simulink model "PVRobusMPC_final"  (R2018a)
settings: Solver=ode2  StartTime=0.0  StopTime=43200  FixedStep=1  RelTol=1e-3  EnableMultiTasking=on
InitFcn:
  | load PV_model_data
StopFcn:
  | save results Lambda_UV01 T_PV_Reference Tm_f01 Pout01 Tamb Time
  | clear all
  | load results
  | figure
  | subplot(3,1,1)
  | plot(Time./3600,T_PV_Reference,Time./3600,Tm_f01)
  | legend('PV Temperature Reference','PV Temperature')
  | title('MPC Tracking')
  | ylim([350 380])
  | subplot(3,1,2)
  | plot(Time./3600,Lambda_UV01)
  | ylim([250 450])
  | legend('\lambda_U_V')
  | subplot(3,1,3)
  | plot(Time./3600,Pout01)
  | legend('PV Power')
  | xlabel('Time [hours]')
  | ylabel('Watt')
values from neighbouring files (symbols this model uses):
  Global_tilt_Irr_2_2_12_13_5 = [0.000279 0.000786 0.00115 0.00401 0.0047 0.0102 0.011 0.0195 0.0266 0.0299 0.0338 0.0682 ... (2802 elements, 1401x2)]    [PV_model_data.mat]
  Total_light_absorption_in_polystyren = [0.0148235487596 0.0159326919994 0.0170383922491 0.0181406655151 0.0192395277052 0.0203349946285 0.0214270819969 0.0225158054254 0.0236011804327 0.0246832224425 0.0257619467839 0.0264640052027 ... (1151 elements, 1151x1)]    [PV_model_data.mat]
  Total_light_absorption_in_PV_cell_acrylic = [0.0222539070262 0.0239185757929 0.0255780524095 0.0272323791236 0.0288816001883 0.030525761736 0.0321649116541 0.0337990994657 0.0354283762117 0.0370527943369 0.0386724075795 0.0397267002838 ... (1151 elements, 1151x1)]    [PV_model_data.mat]
libraries: mpclib x256
(part 60 of 72)

== matlab function PVRobusMPC_final/4 x 4 x 4 PV Panel 4/4 x 4 PV Panel 5/4 PV Panel 1/PV Panel 2/Photovolatic Panel/PV_Cell_Model ==
  data: Total_light_absorption_in_PV_cell_acrylic parameter; Global_tilt_Irr_2_2_12_13_5 parameter; Total_light_absorption_in_polystyren parameter; Tm_i input; Lambda_UV input; Lambda_IR input; Time input; Tm_f output size=1; QQ output; Tambient input; WS input; VL output
function [Tm_f, QQ, VL] = fcn(Total_light_absorption_in_PV_cell_acrylic, Global_tilt_Irr_2_2_12_13_5, Total_light_absorption_in_polystyren, Tm_i, Lambda_UV, Lambda_IR, Time,Tambient,WS)

IL1 = zeros(1,11);
IL1 = IL1';
LambdaIR_Index = 0;
LambdaUV_Index = 0;
Tm_f =0;
temp_out = 0;

k=1.38e-23; %Boltzman constat J/K
h=6.62617e-34; %Planck constant J.s 
c=3e8; %(m/s) light speed
q=1.60218e-19; %(J) charge of electron
Aj= 148.25; % (cm^2)Junction Area calculated from the dimensions of the module, where length*wedth are 125*125 mm2
M= 4; % number of cells in the BP585 module  From area of module divided by area of one cell
A1=(25.6)^2*1e-4; % Whole area of the module in m^2 (26.1 cm by 26.1 cm)
A=M*Aj*1e-4; % (m^2)Area of the module covered with PV cells 
Beta=pi*65/180; % (deg) tilt angle
segma=5.669*10^(-8); %Stefan_Boltzman W/(m^2K^4)
e_sky_clear = 0.95; %emissivity of the sky in clear wheather conditions
e_g = 0.95; % emissivity of the ground
e_m=0.94; %emissivity of the module which is equale to the emissivity of acrylic and glass
deltT=20; % for clear conditions
dt=1; % Define the step value,
K=Time; % constant equal to the number of seconds of sun exposure, this is equivalent to about 18 mins of sun exposure to same (assumed) solar irraiance 
 
%% Calculating the reference saturation current Ior from the unloaded PV module measurements

Voc = 2.084;	%(V) at reference temperature 26.5 C on 02/02 Module 2 with Acrylic
Isc =4.28; % (A)at reference temperature 26.5 C on 02/02 Module 2 with Acrylic
Rch = Voc/Isc; % (Ohm) Characteristic resistance, this should be found at the characteristic Voc and Isc (ex. Temp = 26.5)
N =1.3812; % Ideality factor for Si-Monocrystalline (reference)
Rs= 0.0377; % (Ohm) Series resistance estimated from the IV curve of M2 covered by accrylic
Tmr = 69.5+273.5; %(K) reference temperature
Ior= Isc/(exp(q*Voc/(M*k*N*Tmr))-1); % (A)Reference saturation current
Eg = 1.12; % (eV) bandgap energy of Si

%% Calculating the heat capacity of the module layers

C_PV=A*2330*677*2e-4; % Heat capacity of the cells (equale to area*raw* specific heat*thickness) source: matweb.com
C_Polystyrene= A*1300*121.7*5e-3; %Heat capacity of the Polystyrene Back supporting board to PV cells 
C_acrylic=A*1470*1190*3.2e-3;% Heat capacity of the Acrylic face over the module

Cm=C_PV+C_Polystyrene+C_acrylic; % Heat capacity of the PV module covered with acrylic


if Lambda_IR<300
    Lambda_IR=300;
elseif Lambda_IR>1700
    Lambda_IR=1700;
end

if Lambda_UV<300
    Lambda_UV=300;
elseif Lambda_UV>1700
    Lambda_UV=1700;
end

 LambdaIR_Index=interp1(Global_tilt_Irr_2_2_12_13_5(:,2),1:1401,Lambda_IR,'nearest');
 LambdaUV_Index=interp1(Global_tilt_Irr_2_2_12_13_5(:,2),1:1401,Lambda_UV,'nearest');

%         LambdaIR_Index=j;
%     end
%     if Lambda_UV==Global_tilt_Irr_2_2_12_13_5(j,2)
%         LambdaUV_Index=j;
%     end
% end


 %% Defining the optical and electrical properties of the used PV module
    U= LambdaIR_Index; %Index for Max. wavelength of IR not to block
%     O=1; % Factor to change the ambient temperauter, this is used to factor Taminet (assumable)to vary the reagion. 
    P=1; % P is assumed number of periods that solar irrandiance is almost same for these periods. 
    Index=0; % the index to take off from maximum Lambda IR that can be absorbed
    D=LambdaUV_Index;%1; % initial value that should be given to D (Index for Max. wavelength of UV to block) 
    Lamda = LambdaIR_Index; % 811; % index at which the maximum absorbed wavelength   
    IQE = 0.69005; % internal quantum efficiency of the cell
    RL = 0.356; % (Ohm) Resistive load (designed and experimentally measured)
    IL1(1,1) = 4;% (A) Load current (experimentally measure)
     
%     Lamda
%% Initializing the matrices

%      Io = NaN;
     wavelength=ones(1451,1);
     Tran = ones(1451,1);
     E=ones(1451,1);
     Photon_flux = ones(1451,1);
     Jph=ones(1451,1);
     Iph = ones(1451,1);
%      Voc = ones;
%      IL = ones;
%      VL = ones;
%      P_out = ones;
     frr =ones(1451,1);
     frr_poly = ones(1451,1);
%      Tm=ones(1,D);
%      hc_free=ones(1,D);
     

IL1(1,1) = 4;% (A) Load current (experimentally measure)

%% Finding the phtonic flux
Tran=Total_light_absorption_in_PV_cell_acrylic(1:U); % Total light transmission considering all layers and bounces through them
wavelength= 1e-9.*Global_tilt_Irr_2_2_12_13_5(1:U,2); % (m) wavelength
E = c.*h./wavelength; % (J) Energy per each wavelength
Photon_flux = Global_tilt_Irr_2_2_12_13_5(1:U,1)./E; % (photons/m2/nm/s) photon flux 

% for w=1 %:1:P*K/dt  
   w=1;

   
    Jph(D:Lamda)= q.*Tran(D:1:Lamda).*Photon_flux(D:Lamda).*IQE; %(Culomb/m2/nm/m/s = A/m2/nm)Short circuit current density 
    Iph(D:Lamda)= Aj.*1e-4.*Jph(D:Lamda); % (A/nm) Photo_generated current 


%% Photonic current per one cell
%    for z=D:1:Lamda
%     Jph(z,1)= q*Tran(z,1)*Photon_flux(z,1)*IQE; %(Culomb/m2/nm/m/s = A/m2/nm)Short circuit current density 
%     Iph (z,1) = Aj*1e-4*Jph(z,1); % (A/nm) Photo_generated current 
%    end
  
  Iph_total =0; % Intializing the current
  
%     for j=D:1:Lamda
        Iph_total = sum(Iph(D:Lamda,1)); % (A) Photonic current
%     end    
  
%% Calculating the input power term to cells
      Irr_total=0;
      
%       for j=D:1:Lamda
           E(D:1:Lamda)=h.*c./(wavelength(D:1:Lamda)); %(J) energy in each wavelength
           Irr_total= sum(Photon_flux(D:1:Lamda,1).*E(D:1:Lamda,1));% (W/m2/nm)Irradiance
%            Irr_total= frr(j,1)+Irr_total; % (W/m^2), this represents the integration to calculate total Irradiance for the specific wavelenght range. 
%       end

      Pin=Irr_total* A; % input power (W) to the module of M cells, each has Aj area in cm^2, A=M*Aj*1e-4    
      
%% Calculating the power input to the Polystyrene backing board
    Irr_poly=0;
    
%     for j=D:1:U % This represents the part of the board covered with cell
         E(D:1:U)=h.*c/(wavelength(D:1:U));
%          frr_poly(j,1)=Photon_flux(j,1)*Total_light_absorption_in_polystyren(j,1)*E(j,1);
         Irr_poly=sum(Photon_flux(D:1:U).*Total_light_absorption_in_polystyren(D:1:U).*E(D:1:U));
%     end

    Ppoly =Irr_poly*(A1-A); % (W) The power produced by the light absorbed by the backing Polystyrene plate

%% Calculating the saturation current using the refernece saturation current method
  
Io= Ior * (Tm_i/Tmr)^3*exp(q*Eg*(1/Tmr-1/Tm_i)/(k*N)); %(A) Saturation current as function of temperature
    
%% Calculating the output power consumed by the load
    nu=0.2; % solver constant
    %This loop is to solve for the load current numberically using Euler method 
    for s=1:1:10% s is counter reflects number of the solver steps needed to reach steady state current at a specific time step
        IL1(s+1) =nu*IL1(s)+(1-nu)*( N*k*Tm_i/(q*(RL/M+Rs))*log((Iph_total-IL1(s))/(Io)+1));
    end
%     IL1
    IL = IL1(end); % (V) Stabalized Output current passes the resistive load (0.3525 Ohm)in one time step
%     IL1 = IL1(end);  % setting a new initial load current for the next time step
    VL =  IL *RL; %Load voltage, or Iph_total-Io(w,1)*(exp(q*VL(w,1)/(N*k*Tm(w,1))-1)); %(A) Output current
   
%     P_out =real(VL*IL); %(W) Output power across the load 
   P_out=real(VL*IL);
   P_out=P_out(1);
   QQ=VL.*IL;
%  P_out(w,1)=0; % In case of open circuit condition

%% Calculating the output power in case of tracking the MPP
%      
%      Voc(w,1) = N*k*Tm(w,1)/q*log(Iph_total/Io(w,1)+1) ;  % (V) open circuit voltage
% 
%      Vocn(w,1)=q/(N*k*Tm(w,1))*Voc(w,1); % Normalized open circuit voltage
% 
%      Cff (w,1) = (Vocn(w,1)-log(Vocn(w,1)+0.72))/(Vocn(w,1)+1); % Filling factor
%               
%      rs=Rs/Rch; % ratio
%      
%      Cffn(w,1)=Cff(w,1)*(1-rs); % impact of the series resistance on the IV curve
%      
%     P_out(w,1)=M*Cffn(w,1)*Iph_total*Voc(w,1); % (W) output power of the module
      
%% Defining the terms of heat transfer


 
  hc_forced = 3.3*WS+6.5; % (W/(m^2.K)) Sharples windward relation to calculated hc_forced from the averaged wind speed 
    
  hc_free=1.31*(Tm_i-Tambient)^(1/3); % (W/(M^2.K)) Heat transfer coefficient due to air cooling on top surface and no wind
     
    Tsky=Tambient-deltT; % (K) Sky temperature
    %Tsky=Tambient; % (K) for overcast conditions
    Tground=Tambient; %(K) Ground temperature
     
%% Solving the 1st order nonlinear differenctial equation using Euler method
     Tm_f=Tm_i+dt.*(1/Cm*(segma*A*(((1+cos(Beta)/2)*e_sky_clear*(Tsky)^(4))+((1-cos(Beta))/2*e_g*(Tground)^(4))-(e_m*(Tm_i)^(4)))+ Ppoly + Pin -P_out-A.*(hc_forced^3+hc_free^3).^(1/3).*(Tm_i-Tambient))); %(K)Finding the module Temp

== matlab function PVRobusMPC_final/4 x 4 x 4 PV Panel 4/4 x 4 PV Panel 5/4 PV Panel 1/PV Panel 3/Photovolatic Panel/PV_Cell_Model ==
  data: Total_light_absorption_in_PV_cell_acrylic parameter; Global_tilt_Irr_2_2_12_13_5 parameter; Total_light_absorption_in_polystyren parameter; Tm_i input; Lambda_UV input; Lambda_IR input; Time input; Tm_f output size=1; QQ output; Tambient input; WS input; VL output
function [Tm_f, QQ, VL] = fcn(Total_light_absorption_in_PV_cell_acrylic, Global_tilt_Irr_2_2_12_13_5, Total_light_absorption_in_polystyren, Tm_i, Lambda_UV, Lambda_IR, Time,Tambient,WS)

IL1 = zeros(1,11);
IL1 = IL1';
LambdaIR_Index = 0;
LambdaUV_Index = 0;
Tm_f =0;
temp_out = 0;

k=1.38e-23; %Boltzman constat J/K
h=6.62617e-34; %Planck constant J.s 
c=3e8; %(m/s) light speed
q=1.60218e-19; %(J) charge of electron
Aj= 148.25; % (cm^2)Junction Area calculated from the dimensions of the module, where length*wedth are 125*125 mm2
M= 4; % number of cells in the BP585 module  From area of module divided by area of one cell
A1=(25.6)^2*1e-4; % Whole area of the module in m^2 (26.1 cm by 26.1 cm)
A=M*Aj*1e-4; % (m^2)Area of the module covered with PV cells 
Beta=pi*65/180; % (deg) tilt angle
segma=5.669*10^(-8); %Stefan_Boltzman W/(m^2K^4)
e_sky_clear = 0.95; %emissivity of the sky in clear wheather conditions
e_g = 0.95; % emissivity of the ground
e_m=0.94; %emissivity of the module which is equale to the emissivity of acrylic and glass
deltT=20; % for clear conditions
dt=1; % Define the step value,
K=Time; % constant equal to the number of seconds of sun exposure, this is equivalent to about 18 mins of sun exposure to same (assumed) solar irraiance 
 
%% Calculating the reference saturation current Ior from the unloaded PV module measurements

Voc = 2.084;	%(V) at reference temperature 26.5 C on 02/02 Module 2 with Acrylic
Isc =4.28; % (A)at reference temperature 26.5 C on 02/02 Module 2 with Acrylic
Rch = Voc/Isc; % (Ohm) Characteristic resistance, this should be found at the characteristic Voc and Isc (ex. Temp = 26.5)
N =1.3812; % Ideality factor for Si-Monocrystalline (reference)
Rs= 0.0377; % (Ohm) Series resistance estimated from the IV curve of M2 covered by accrylic
Tmr = 69.5+273.5; %(K) reference temperature
Ior= Isc/(exp(q*Voc/(M*k*N*Tmr))-1); % (A)Reference saturation current
Eg = 1.12; % (eV) bandgap energy of Si

%% Calculating the heat capacity of the module layers

C_PV=A*2330*677*2e-4; % Heat capacity of the cells (equale to area*raw* specific heat*thickness) source: matweb.com
C_Polystyrene= A*1300*121.7*5e-3; %Heat capacity of the Polystyrene Back supporting board to PV cells 
C_acrylic=A*1470*1190*3.2e-3;% Heat capacity of the Acrylic face over the module

Cm=C_PV+C_Polystyrene+C_acrylic; % Heat capacity of the PV module covered with acrylic


if Lambda_IR<300
    Lambda_IR=300;
elseif Lambda_IR>1700
    Lambda_IR=1700;
end

if Lambda_UV<300
    Lambda_UV=300;
elseif Lambda_UV>1700
    Lambda_UV=1700;
end

 LambdaIR_Index=interp1(Global_tilt_Irr_2_2_12_13_5(:,2),1:1401,Lambda_IR,'nearest');
 LambdaUV_Index=interp1(Global_tilt_Irr_2_2_12_13_5(:,2),1:1401,Lambda_UV,'nearest');

%         LambdaIR_Index=j;
%     end
%     if Lambda_UV==Global_tilt_Irr_2_2_12_13_5(j,2)
%         LambdaUV_Index=j;
%     end
% end


 %% Defining the optical and electrical properties of the used PV module
    U= LambdaIR_Index; %Index for Max. wavelength of IR not to block
%     O=1; % Factor to change the ambient temperauter, this is used to factor Taminet (assumable)to vary the reagion. 
    P=1; % P is assumed number of periods that solar irrandiance is almost same for these periods. 
    Index=0; % the index to take off from maximum Lambda IR that can be absorbed
    D=LambdaUV_Index;%1; % initial value that should be given to D (Index for Max. wavelength of UV to block) 
    Lamda = LambdaIR_Index; % 811; % index at which the maximum absorbed wavelength   
    IQE = 0.69005; % internal quantum efficiency of the cell
    RL = 0.356; % (Ohm) Resistive load (designed and experimentally measured)
    IL1(1,1) = 4;% (A) Load current (experimentally measure)
     
%     Lamda
%% Initializing the matrices

%      Io = NaN;
     wavelength=ones(1451,1);
     Tran = ones(1451,1);
     E=ones(1451,1);
     Photon_flux = ones(1451,1);
     Jph=ones(1451,1);
     Iph = ones(1451,1);
%      Voc = ones;
%      IL = ones;
%      VL = ones;
%      P_out = ones;
     frr =ones(1451,1);
     frr_poly = ones(1451,1);
%      Tm=ones(1,D);
%      hc_free=ones(1,D);
     

IL1(1,1) = 4;% (A) Load current (experimentally measure)

%% Finding the phtonic flux
Tran=Total_light_absorption_in_PV_cell_acrylic(1:U); % Total light transmission considering all layers and bounces through them
wavelength= 1e-9.*Global_tilt_Irr_2_2_12_13_5(1:U,2); % (m) wavelength
E = c.*h./wavelength; % (J) Energy per each wavelength
Photon_flux = Global_tilt_Irr_2_2_12_13_5(1:U,1)./E; % (photons/m2/nm/s) photon flux 

% for w=1 %:1:P*K/dt  
   w=1;

   
    Jph(D:Lamda)= q.*Tran(D:1:Lamda).*Photon_flux(D:Lamda).*IQE; %(Culomb/m2/nm/m/s = A/m2/nm)Short circuit current density 
    Iph(D:Lamda)= Aj.*1e-4.*Jph(D:Lamda); % (A/nm) Photo_generated current 


%% Photonic current per one cell
%    for z=D:1:Lamda
%     Jph(z,1)= q*Tran(z,1)*Photon_flux(z,1)*IQE; %(Culomb/m2/nm/m/s = A/m2/nm)Short circuit current density 
%     Iph (z,1) = Aj*1e-4*Jph(z,1); % (A/nm) Photo_generated current 
%    end
  
  Iph_total =0; % Intializing the current
  
%     for j=D:1:Lamda
        Iph_total = sum(Iph(D:Lamda,1)); % (A) Photonic current
%     end    
  
%% Calculating the input power term to cells
      Irr_total=0;
      
%       for j=D:1:Lamda
           E(D:1:Lamda)=h.*c./(wavelength(D:1:Lamda)); %(J) energy in each wavelength
           Irr_total= sum(Photon_flux(D:1:Lamda,1).*E(D:1:Lamda,1));% (W/m2/nm)Irradiance
%            Irr_total= frr(j,1)+Irr_total; % (W/m^2), this represents the integration to calculate total Irradiance for the specific wavelenght range. 
%       end

      Pin=Irr_total* A; % input power (W) to the module of M cells, each has Aj area in cm^2, A=M*Aj*1e-4    
      
%% Calculating the power input to the Polystyrene backing board
    Irr_poly=0;
    
%     for j=D:1:U % This represents the part of the board covered with cell
         E(D:1:U)=h.*c/(wavelength(D:1:U));
%          frr_poly(j,1)=Photon_flux(j,1)*Total_light_absorption_in_polystyren(j,1)*E(j,1);
         Irr_poly=sum(Photon_flux(D:1:U).*Total_light_absorption_in_polystyren(D:1:U).*E(D:1:U));
%     end

    Ppoly =Irr_poly*(A1-A); % (W) The power produced by the light absorbed by the backing Polystyrene plate

%% Calculating the saturation current using the refernece saturation current method
  
Io= Ior * (Tm_i/Tmr)^3*exp(q*Eg*(1/Tmr-1/Tm_i)/(k*N)); %(A) Saturation current as function of temperature
    
%% Calculating the output power consumed by the load
    nu=0.2; % solver constant
    %This loop is to solve for the load current numberically using Euler method 
    for s=1:1:10% s is counter reflects number of the solver steps needed to reach steady state current at a specific time step
        IL1(s+1) =nu*IL1(s)+(1-nu)*( N*k*Tm_i/(q*(RL/M+Rs))*log((Iph_total-IL1(s))/(Io)+1));
    end
%     IL1
    IL = IL1(end); % (V) Stabalized Output current passes the resistive load (0.3525 Ohm)in one time step
%     IL1 = IL1(end);  % setting a new initial load current for the next time step
    VL =  IL *RL; %Load voltage, or Iph_total-Io(w,1)*(exp(q*VL(w,1)/(N*k*Tm(w,1))-1)); %(A) Output current
   
%     P_out =real(VL*IL); %(W) Output power across the load 
   P_out=real(VL*IL);
   P_out=P_out(1);
   QQ=VL.*IL;
%  P_out(w,1)=0; % In case of open circuit condition

%% Calculating the output power in case of tracking the MPP
%      
%      Voc(w,1) = N*k*Tm(w,1)/q*log(Iph_total/Io(w,1)+1) ;  % (V) open circuit voltage
% 
%      Vocn(w,1)=q/(N*k*Tm(w,1))*Voc(w,1); % Normalized open circuit voltage
% 
%      Cff (w,1) = (Vocn(w,1)-log(Vocn(w,1)+0.72))/(Vocn(w,1)+1); % Filling factor
%               
%      rs=Rs/Rch; % ratio
%      
%      Cffn(w,1)=Cff(w,1)*(1-rs); % impact of the series resistance on the IV curve
%      
%     P_out(w,1)=M*Cffn(w,1)*Iph_total*Voc(w,1); % (W) output power of the module
      
%% Defining the terms of heat transfer


 
  hc_forced = 3.3*WS+6.5; % (W/(m^2.K)) Sharples windward relation to calculated hc_forced from the averaged wind speed 
    
  hc_free=1.31*(Tm_i-Tambient)^(1/3); % (W/(M^2.K)) Heat transfer coefficient due to air cooling on top surface and no wind
     
    Tsky=Tambient-deltT; % (K) Sky temperature
    %Tsky=Tambient; % (K) for overcast conditions
    Tground=Tambient; %(K) Ground temperature
     
%% Solving the 1st order nonlinear differenctial equation using Euler method
     Tm_f=Tm_i+dt.*(1/Cm*(segma*A*(((1+cos(Beta)/2)*e_sky_clear*(Tsky)^(4))+((1-cos(Beta))/2*e_g*(Tground)^(4))-(e_m*(Tm_i)^(4)))+ Ppoly + Pin -P_out-A.*(hc_forced^3+hc_free^3).^(1/3).*(Tm_i-Tambient))); %(K)Finding the module Temp

== matlab function PVRobusMPC_final/4 x 4 x 4 PV Panel 4/4 x 4 PV Panel 5/4 PV Panel 1/PV Panel 4/Photovolatic Panel/PV_Cell_Model ==
  data: Total_light_absorption_in_PV_cell_acrylic parameter; Global_tilt_Irr_2_2_12_13_5 parameter; Total_light_absorption_in_polystyren parameter; Tm_i input; Lambda_UV input; Lambda_IR input; Time input; Tm_f output size=1; QQ output; Tambient input; WS input; VL output
function [Tm_f, QQ, VL] = fcn(Total_light_absorption_in_PV_cell_acrylic, Global_tilt_Irr_2_2_12_13_5, Total_light_absorption_in_polystyren, Tm_i, Lambda_UV, Lambda_IR, Time,Tambient,WS)

IL1 = zeros(1,11);
IL1 = IL1';
LambdaIR_Index = 0;
LambdaUV_Index = 0;
Tm_f =0;
temp_out = 0;

k=1.38e-23; %Boltzman constat J/K
h=6.62617e-34; %Planck constant J.s 
c=3e8; %(m/s) light speed
q=1.60218e-19; %(J) charge of electron
Aj= 148.25; % (cm^2)Junction Area calculated from the dimensions of the module, where length*wedth are 125*125 mm2
M= 4; % number of cells in the BP585 module  From area of module divided by area of one cell
A1=(25.6)^2*1e-4; % Whole area of the module in m^2 (26.1 cm by 26.1 cm)
A=M*Aj*1e-4; % (m^2)Area of the module covered with PV cells 
Beta=pi*65/180; % (deg) tilt angle
segma=5.669*10^(-8); %Stefan_Boltzman W/(m^2K^4)
e_sky_clear = 0.95; %emissivity of the sky in clear wheather conditions
e_g = 0.95; % emissivity of the ground
e_m=0.94; %emissivity of the module which is equale to the emissivity of acrylic and glass
deltT=20; % for clear conditions
dt=1; % Define the step value,
K=Time; % constant equal to the number of seconds of sun exposure, this is equivalent to about 18 mins of sun exposure to same (assumed) solar irraiance 
 
%% Calculating the reference saturation current Ior from the unloaded PV module measurements

Voc = 2.084;	%(V) at reference temperature 26.5 C on 02/02 Module 2 with Acrylic
Isc =4.28; % (A)at reference temperature 26.5 C on 02/02 Module 2 with Acrylic
Rch = Voc/Isc; % (Ohm) Characteristic resistance, this should be found at the characteristic Voc and Isc (ex. Temp = 26.5)
N =1.3812; % Ideality factor for Si-Monocrystalline (reference)
Rs= 0.0377; % (Ohm) Series resistance estimated from the IV curve of M2 covered by accrylic
Tmr = 69.5+273.5; %(K) reference temperature
Ior= Isc/(exp(q*Voc/(M*k*N*Tmr))-1); % (A)Reference saturation current
Eg = 1.12; % (eV) bandgap energy of Si

%% Calculating the heat capacity of the module layers

C_PV=A*2330*677*2e-4; % Heat capacity of the cells (equale to area*raw* specific heat*thickness) source: matweb.com
C_Polystyrene= A*1300*121.7*5e-3; %Heat capacity of the Polystyrene Back supporting board to PV cells 
C_acrylic=A*1470*1190*3.2e-3;% Heat capacity of the Acrylic face over the module

Cm=C_PV+C_Polystyrene+C_acrylic; % Heat capacity of the PV module covered with acrylic


if Lambda_IR<300
    Lambda_IR=300;
elseif Lambda_IR>1700
    Lambda_IR=1700;
end

if Lambda_UV<300
    Lambda_UV=300;
elseif Lambda_UV>1700
    Lambda_UV=1700;
end

 LambdaIR_Index=interp1(Global_tilt_Irr_2_2_12_13_5(:,2),1:1401,Lambda_IR,'nearest');
 LambdaUV_Index=interp1(Global_tilt_Irr_2_2_12_13_5(:,2),1:1401,Lambda_UV,'nearest');

%         LambdaIR_Index=j;
%     end
%     if Lambda_UV==Global_tilt_Irr_2_2_12_13_5(j,2)
%         LambdaUV_Index=j;
%     end
% end


 %% Defining the optical and electrical properties of the used PV module
    U= LambdaIR_Index; %Index for Max. wavelength of IR not to block
%     O=1; % Factor to change the ambient temperauter, this is used to factor Taminet (assumable)to vary the reagion. 
    P=1; % P is assumed number of periods that solar irrandiance is almost same for these periods. 
    Index=0; % the index to take off from maximum Lambda IR that can be absorbed
    D=LambdaUV_Index;%1; % initial value that should be given to D (Index for Max. wavelength of UV to block) 
    Lamda = LambdaIR_Index; % 811; % index at which the maximum absorbed wavelength   
    IQE = 0.69005; % internal quantum efficiency of the cell
    RL = 0.356; % (Ohm) Resistive load (designed and experimentally measured)
    IL1(1,1) = 4;% (A) Load current (experimentally measure)
     
%     Lamda
%% Initializing the matrices

%      Io = NaN;
     wavelength=ones(1451,1);
     Tran = ones(1451,1);
     E=ones(1451,1);
     Photon_flux = ones(1451,1);
     Jph=ones(1451,1);
     Iph = ones(1451,1);
%      Voc = ones;
%      IL = ones;
%      VL = ones;
%      P_out = ones;
     frr =ones(1451,1);
     frr_poly = ones(1451,1);
%      Tm=ones(1,D);
%      hc_free=ones(1,D);
     

IL1(1,1) = 4;% (A) Load current (experimentally measure)

%% Finding the phtonic flux
Tran=Total_light_absorption_in_PV_cell_acrylic(1:U); % Total light transmission considering all layers and bounces through them
wavelength= 1e-9.*Global_tilt_Irr_2_2_12_13_5(1:U,2); % (m) wavelength
E = c.*h./wavelength; % (J) Energy per each wavelength
Photon_flux = Global_tilt_Irr_2_2_12_13_5(1:U,1)./E; % (photons/m2/nm/s) photon flux 

% for w=1 %:1:P*K/dt  
   w=1;

   
    Jph(D:Lamda)= q.*Tran(D:1:Lamda).*Photon_flux(D:Lamda).*IQE; %(Culomb/m2/nm/m/s = A/m2/nm)Short circuit current density 
    Iph(D:Lamda)= Aj.*1e-4.*Jph(D:Lamda); % (A/nm) Photo_generated current 


%% Photonic current per one cell
%    for z=D:1:Lamda
%     Jph(z,1)= q*Tran(z,1)*Photon_flux(z,1)*IQE; %(Culomb/m2/nm/m/s = A/m2/nm)Short circuit current density 
%     Iph (z,1) = Aj*1e-4*Jph(z,1); % (A/nm) Photo_generated current 
%    end
  
  Iph_total =0; % Intializing the current
  
%     for j=D:1:Lamda
        Iph_total = sum(Iph(D:Lamda,1)); % (A) Photonic current
%     end    
  
%% Calculating the input power term to cells
      Irr_total=0;
      
%       for j=D:1:Lamda
           E(D:1:Lamda)=h.*c./(wavelength(D:1:Lamda)); %(J) energy in each wavelength
           Irr_total= sum(Photon_flux(D:1:Lamda,1).*E(D:1:Lamda,1));% (W/m2/nm)Irradiance
%            Irr_total= frr(j,1)+Irr_total; % (W/m^2), this represents the integration to calculate total Irradiance for the specific wavelenght range. 
%       end

      Pin=Irr_total* A; % input power (W) to the module of M cells, each has Aj area in cm^2, A=M*Aj*1e-4    
      
%% Calculating the power input to the Polystyrene backing board
    Irr_poly=0;
    
%     for j=D:1:U % This represents the part of the board covered with cell
         E(D:1:U)=h.*c/(wavelength(D:1:U));
%          frr_poly(j,1)=Photon_flux(j,1)*Total_light_absorption_in_polystyren(j,1)*E(j,1);
         Irr_poly=sum(Photon_flux(D:1:U).*Total_light_absorption_in_polystyren(D:1:U).*E(D:1:U));
%     end

    Ppoly =Irr_poly*(A1-A); % (W) The power produced by the light absorbed by the backing Polystyrene plate

%% Calculating the saturation current using the refernece saturation current method
  
Io= Ior * (Tm_i/Tmr)^3*exp(q*Eg*(1/Tmr-1/Tm_i)/(k*N)); %(A) Saturation current as function of temperature
    
%% Calculating the output power consumed by the load
    nu=0.2; % solver constant
    %This loop is to solve for the load current numberically using Euler method 
    for s=1:1:10% s is counter reflects number of the solver steps needed to reach steady state current at a specific time step
        IL1(s+1) =nu*IL1(s)+(1-nu)*( N*k*Tm_i/(q*(RL/M+Rs))*log((Iph_total-IL1(s))/(Io)+1));
    end
%     IL1
    IL = IL1(end); % (V) Stabalized Output current passes the resistive load (0.3525 Ohm)in one time step
%     IL1 = IL1(end);  % setting a new initial load current for the next time step
    VL =  IL *RL; %Load voltage, or Iph_total-Io(w,1)*(exp(q*VL(w,1)/(N*k*Tm(w,1))-1)); %(A) Output current
   
%     P_out =real(VL*IL); %(W) Output power across the load 
   P_out=real(VL*IL);
   P_out=P_out(1);
   QQ=VL.*IL;
%  P_out(w,1)=0; % In case of open circuit condition

%% Calculating the output power in case of tracking the MPP
%      
%      Voc(w,1) = N*k*Tm(w,1)/q*log(Iph_total/Io(w,1)+1) ;  % (V) open circuit voltage
% 
%      Vocn(w,1)=q/(N*k*Tm(w,1))*Voc(w,1); % Normalized open circuit voltage
% 
%      Cff (w,1) = (Vocn(w,1)-log(Vocn(w,1)+0.72))/(Vocn(w,1)+1); % Filling factor
%               
%      rs=Rs/Rch; % ratio
%      
%      Cffn(w,1)=Cff(w,1)*(1-rs); % impact of the series resistance on the IV curve
%      
%     P_out(w,1)=M*Cffn(w,1)*Iph_total*Voc(w,1); % (W) output power of the module
      
%% Defining the terms of heat transfer


 
  hc_forced = 3.3*WS+6.5; % (W/(m^2.K)) Sharples windward relation to calculated hc_forced from the averaged wind speed 
    
  hc_free=1.31*(Tm_i-Tambient)^(1/3); % (W/(M^2.K)) Heat transfer coefficient due to air cooling on top surface and no wind
     
    Tsky=Tambient-deltT; % (K) Sky temperature
    %Tsky=Tambient; % (K) for overcast conditions
    Tground=Tambient; %(K) Ground temperature
     
%% Solving the 1st order nonlinear differenctial equation using Euler method
     Tm_f=Tm_i+dt.*(1/Cm*(segma*A*(((1+cos(Beta)/2)*e_sky_clear*(Tsky)^(4))+((1-cos(Beta))/2*e_g*(Tground)^(4))-(e_m*(Tm_i)^(4)))+ Ppoly + Pin -P_out-A.*(hc_forced^3+hc_free^3).^(1/3).*(Tm_i-Tambient))); %(K)Finding the module Temp

== matlab function PVRobusMPC_final/4 x 4 x 4 PV Panel 4/4 x 4 PV Panel 5/4 PV Panel 2/PV Panel 5/Photovolatic Panel/PV_Cell_Model ==
  data: Total_light_absorption_in_PV_cell_acrylic parameter; Global_tilt_Irr_2_2_12_13_5 parameter; Total_light_absorption_in_polystyren parameter; Tm_i input; Lambda_UV input; Lambda_IR input; Time input; Tm_f output size=1; QQ output; Tambient input; WS input; VL output
function [Tm_f, QQ, VL] = fcn(Total_light_absorption_in_PV_cell_acrylic, Global_tilt_Irr_2_2_12_13_5, Total_light_absorption_in_polystyren, Tm_i, Lambda_UV, Lambda_IR, Time,Tambient,WS)

IL1 = zeros(1,11);
IL1 = IL1';
LambdaIR_Index = 0;
LambdaUV_Index = 0;
Tm_f =0;
temp_out = 0;

k=1.38e-23; %Boltzman constat J/K
h=6.62617e-34; %Planck constant J.s 
c=3e8; %(m/s) light speed
q=1.60218e-19; %(J) charge of electron
Aj= 148.25; % (cm^2)Junction Area calculated from the dimensions of the module, where length*wedth are 125*125 mm2
M= 4; % number of cells in the BP585 module  From area of module divided by area of one cell
A1=(25.6)^2*1e-4; % Whole area of the module in m^2 (26.1 cm by 26.1 cm)
A=M*Aj*1e-4; % (m^2)Area of the module covered with PV cells 
Beta=pi*65/180; % (deg) tilt angle
segma=5.669*10^(-8); %Stefan_Boltzman W/(m^2K^4)
e_sky_clear = 0.95; %emissivity of the sky in clear wheather conditions
e_g = 0.95; % emissivity of the ground
e_m=0.94; %emissivity of the module which is equale to the emissivity of acrylic and glass
deltT=20; % for clear conditions
dt=1; % Define the step value,
K=Time; % constant equal to the number of seconds of sun exposure, this is equivalent to about 18 mins of sun exposure to same (assumed) solar irraiance 
 
%% Calculating the reference saturation current Ior from the unloaded PV module measurements

Voc = 2.084;	%(V) at reference temperature 26.5 C on 02/02 Module 2 with Acrylic
Isc =4.28; % (A)at reference temperature 26.5 C on 02/02 Module 2 with Acrylic
Rch = Voc/Isc; % (Ohm) Characteristic resistance, this should be found at the characteristic Voc and Isc (ex. Temp = 26.5)
N =1.3812; % Ideality factor for Si-Monocrystalline (reference)
Rs= 0.0377; % (Ohm) Series resistance estimated from the IV curve of M2 covered by accrylic
Tmr = 69.5+273.5; %(K) reference temperature
Ior= Isc/(exp(q*Voc/(M*k*N*Tmr))-1); % (A)Reference saturation current
Eg = 1.12; % (eV) bandgap energy of Si

%% Calculating the heat capacity of the module layers

C_PV=A*2330*677*2e-4; % Heat capacity of the cells (equale to area*raw* specific heat*thickness) source: matweb.com
C_Polystyrene= A*1300*121.7*5e-3; %Heat capacity of the Polystyrene Back supporting board to PV cells 
C_acrylic=A*1470*1190*3.2e-3;% Heat capacity of the Acrylic face over the module

Cm=C_PV+C_Polystyrene+C_acrylic; % Heat capacity of the PV module covered with acrylic


if Lambda_IR<300
    Lambda_IR=300;
elseif Lambda_IR>1700
    Lambda_IR=1700;
end

if Lambda_UV<300
    Lambda_UV=300;
elseif Lambda_UV>1700
    Lambda_UV=1700;
end

 LambdaIR_Index=interp1(Global_tilt_Irr_2_2_12_13_5(:,2),1:1401,Lambda_IR,'nearest');
 LambdaUV_Index=interp1(Global_tilt_Irr_2_2_12_13_5(:,2),1:1401,Lambda_UV,'nearest');

%         LambdaIR_Index=j;
%     end
%     if Lambda_UV==Global_tilt_Irr_2_2_12_13_5(j,2)
%         LambdaUV_Index=j;
%     end
% end


 %% Defining the optical and electrical properties of the used PV module
    U= LambdaIR_Index; %Index for Max. wavelength of IR not to block
%     O=1; % Factor to change the ambient temperauter, this is used to factor Taminet (assumable)to vary the reagion. 
    P=1; % P is assumed number of periods that solar irrandiance is almost same for these periods. 
    Index=0; % the index to take off from maximum Lambda IR that can be absorbed
    D=LambdaUV_Index;%1; % initial value that should be given to D (Index for Max. wavelength of UV to block) 
    Lamda = LambdaIR_Index; % 811; % index at which the maximum absorbed wavelength   
    IQE = 0.69005; % internal quantum efficiency of the cell
    RL = 0.356; % (Ohm) Resistive load (designed and experimentally measured)
    IL1(1,1) = 4;% (A) Load current (experimentally measure)
     
%     Lamda
%% Initializing the matrices

%      Io = NaN;
     wavelength=ones(1451,1);
     Tran = ones(1451,1);
     E=ones(1451,1);
     Photon_flux = ones(1451,1);
     Jph=ones(1451,1);
     Iph = ones(1451,1);
%      Voc = ones;
%      IL = ones;
%      VL = ones;
%      P_out = ones;
     frr =ones(1451,1);
     frr_poly = ones(1451,1);
%      Tm=ones(1,D);
%      hc_free=ones(1,D);
     

IL1(1,1) = 4;% (A) Load current (experimentally measure)

%% Finding the phtonic flux
Tran=Total_light_absorption_in_PV_cell_acrylic(1:U); % Total light transmission considering all layers and bounces through them
wavelength= 1e-9.*Global_tilt_Irr_2_2_12_13_5(1:U,2); % (m) wavelength
E = c.*h./wavelength; % (J) Energy per each wavelength
Photon_flux = Global_tilt_Irr_2_2_12_13_5(1:U,1)./E; % (photons/m2/nm/s) photon flux 

% for w=1 %:1:P*K/dt  
   w=1;

   
    Jph(D:Lamda)= q.*Tran(D:1:Lamda).*Photon_flux(D:Lamda).*IQE; %(Culomb/m2/nm/m/s = A/m2/nm)Short circuit current density 
    Iph(D:Lamda)= Aj.*1e-4.*Jph(D:Lamda); % (A/nm) Photo_generated current 


%% Photonic current per one cell
%    for z=D:1:Lamda
%     Jph(z,1)= q*Tran(z,1)*Photon_flux(z,1)*IQE; %(Culomb/m2/nm/m/s = A/m2/nm)Short circuit current density 
%     Iph (z,1) = Aj*1e-4*Jph(z,1); % (A/nm) Photo_generated current 
%    end
  
  Iph_total =0; % Intializing the current
  
%     for j=D:1:Lamda
        Iph_total = sum(Iph(D:Lamda,1)); % (A) Photonic current
%     end    
  
%% Calculating the input power term to cells
      Irr_total=0;
      
%       for j=D:1:Lamda
           E(D:1:Lamda)=h.*c./(wavelength(D:1:Lamda)); %(J) energy in each wavelength
           Irr_total= sum(Photon_flux(D:1:Lamda,1).*E(D:1:Lamda,1));% (W/m2/nm)Irradiance
%            Irr_total= frr(j,1)+Irr_total; % (W/m^2), this represents the integration to calculate total Irradiance for the specific wavelenght range. 
%       end

      Pin=Irr_total* A; % input power (W) to the module of M cells, each has Aj area in cm^2, A=M*Aj*1e-4    
      
%% Calculating the power input to the Polystyrene backing board
    Irr_poly=0;
    
%     for j=D:1:U % This represents the part of the board covered with cell
         E(D:1:U)=h.*c/(wavelength(D:1:U));
%          frr_poly(j,1)=Photon_flux(j,1)*Total_light_absorption_in_polystyren(j,1)*E(j,1);
         Irr_poly=sum(Photon_flux(D:1:U).*Total_light_absorption_in_polystyren(D:1:U).*E(D:1:U));
%     end

    Ppoly =Irr_poly*(A1-A); % (W) The power produced by the light absorbed by the backing Polystyrene plate

%% Calculating the saturation current using the refernece saturation current method
  
Io= Ior * (Tm_i/Tmr)^3*exp(q*Eg*(1/Tmr-1/Tm_i)/(k*N)); %(A) Saturation current as function of temperature
    
%% Calculating the output power consumed by the load
    nu=0.2; % solver constant
    %This loop is to solve for the load current numberically using Euler method 
    for s=1:1:10% s is counter reflects number of the solver steps needed to reach steady state current at a specific time step
        IL1(s+1) =nu*IL1(s)+(1-nu)*( N*k*Tm_i/(q*(RL/M+Rs))*log((Iph_total-IL1(s))/(Io)+1));
    end
%     IL1
    IL = IL1(end); % (V) Stabalized Output current passes the resistive load (0.3525 Ohm)in one time step
%     IL1 = IL1(end);  % setting a new initial load current for the next time step
    VL =  IL *RL; %Load voltage, or Iph_total-Io(w,1)*(exp(q*VL(w,1)/(N*k*Tm(w,1))-1)); %(A) Output current
   
%     P_out =real(VL*IL); %(W) Output power across the load 
   P_out=real(VL*IL);
   P_out=P_out(1);
   QQ=VL.*IL;
%  P_out(w,1)=0; % In case of open circuit condition

%% Calculating the output power in case of tracking the MPP
%      
%      Voc(w,1) = N*k*Tm(w,1)/q*log(Iph_total/Io(w,1)+1) ;  % (V) open circuit voltage
% 
%      Vocn(w,1)=q/(N*k*Tm(w,1))*Voc(w,1); % Normalized open circuit voltage
% 
%      Cff (w,1) = (Vocn(w,1)-log(Vocn(w,1)+0.72))/(Vocn(w,1)+1); % Filling factor
%               
%      rs=Rs/Rch; % ratio
%      
%      Cffn(w,1)=Cff(w,1)*(1-rs); % impact of the series resistance on the IV curve
%      
%     P_out(w,1)=M*Cffn(w,1)*Iph_total*Voc(w,1); % (W) output power of the module
      
%% Defining the terms of heat transfer


 
  hc_forced = 3.3*WS+6.5; % (W/(m^2.K)) Sharples windward relation to calculated hc_forced from the averaged wind speed 
    
  hc_free=1.31*(Tm_i-Tambient)^(1/3); % (W/(M^2.K)) Heat transfer coefficient due to air cooling on top surface and no wind
     
    Tsky=Tambient-deltT; % (K) Sky temperature
    %Tsky=Tambient; % (K) for overcast conditions
    Tground=Tambient; %(K) Ground temperature
     
%% Solving the 1st order nonlinear differenctial equation using Euler method
     Tm_f=Tm_i+dt.*(1/Cm*(segma*A*(((1+cos(Beta)/2)*e_sky_clear*(Tsky)^(4))+((1-cos(Beta))/2*e_g*(Tground)^(4))-(e_m*(Tm_i)^(4)))+ Ppoly + Pin -P_out-A.*(hc_forced^3+hc_free^3).^(1/3).*(Tm_i-Tambient))); %(K)Finding the module Temp

== matlab function PVRobusMPC_final/4 x 4 x 4 PV Panel 4/4 x 4 PV Panel 5/4 PV Panel 2/PV Panel 6/Photovolatic Panel/PV_Cell_Model ==
  data: Total_light_absorption_in_PV_cell_acrylic parameter; Global_tilt_Irr_2_2_12_13_5 parameter; Total_light_absorption_in_polystyren parameter; Tm_i input; Lambda_UV input; Lambda_IR input; Time input; Tm_f output size=1; QQ output; Tambient input; WS input; VL output
function [Tm_f, QQ, VL] = fcn(Total_light_absorption_in_PV_cell_acrylic, Global_tilt_Irr_2_2_12_13_5, Total_light_absorption_in_polystyren, Tm_i, Lambda_UV, Lambda_IR, Time,Tambient,WS)

IL1 = zeros(1,11);
IL1 = IL1';
LambdaIR_Index = 0;
LambdaUV_Index = 0;
Tm_f =0;
temp_out = 0;

k=1.38e-23; %Boltzman constat J/K
h=6.62617e-34; %Planck constant J.s 
c=3e8; %(m/s) light speed
q=1.60218e-19; %(J) charge of electron
Aj= 148.25; % (cm^2)Junction Area calculated from the dimensions of the module, where length*wedth are 125*125 mm2
M= 4; % number of cells in the BP585 module  From area of module divided by area of one cell
A1=(25.6)^2*1e-4; % Whole area of the module in m^2 (26.1 cm by 26.1 cm)
A=M*Aj*1e-4; % (m^2)Area of the module covered with PV cells 
Beta=pi*65/180; % (deg) tilt angle
segma=5.669*10^(-8); %Stefan_Boltzman W/(m^2K^4)
e_sky_clear = 0.95; %emissivity of the sky in clear wheather conditions
e_g = 0.95; % emissivity of the ground
e_m=0.94; %emissivity of the module which is equale to the emissivity of acrylic and glass
deltT=20; % for clear conditions
dt=1; % Define the step value,
K=Time; % constant equal to the number of seconds of sun exposure, this is equivalent to about 18 mins of sun exposure to same (assumed) solar irraiance 
 
%% Calculating the reference saturation current Ior from the unloaded PV module measurements

Voc = 2.084;	%(V) at reference temperature 26.5 C on 02/02 Module 2 with Acrylic
Isc =4.28; % (A)at reference temperature 26.5 C on 02/02 Module 2 with Acrylic
Rch = Voc/Isc; % (Ohm) Characteristic resistance, this should be found at the characteristic Voc and Isc (ex. Temp = 26.5)
N =1.3812; % Ideality factor for Si-Monocrystalline (reference)
Rs= 0.0377; % (Ohm) Series resistance estimated from the IV curve of M2 covered by accrylic
Tmr = 69.5+273.5; %(K) reference temperature
Ior= Isc/(exp(q*Voc/(M*k*N*Tmr))-1); % (A)Reference saturation current
Eg = 1.12; % (eV) bandgap energy of Si

%% Calculating the heat capacity of the module layers

C_PV=A*2330*677*2e-4; % Heat capacity of the cells (equale to area*raw* specific heat*thickness) source: matweb.com
C_Polystyrene= A*1300*121.7*5e-3; %Heat capacity of the Polystyrene Back supporting board to PV cells 
C_acrylic=A*1470*1190*3.2e-3;% Heat capacity of the Acrylic face over the module

Cm=C_PV+C_Polystyrene+C_acrylic; % Heat capacity of the PV module covered with acrylic


if Lambda_IR<300
    Lambda_IR=300;
elseif Lambda_IR>1700
    Lambda_IR=1700;
end

if Lambda_UV<300
    Lambda_UV=300;
elseif Lambda_UV>1700
    Lambda_UV=1700;
end

 LambdaIR_Index=interp1(Global_tilt_Irr_2_2_12_13_5(:,2),1:1401,Lambda_IR,'nearest');
 LambdaUV_Index=interp1(Global_tilt_Irr_2_2_12_13_5(:,2),1:1401,Lambda_UV,'nearest');

%         LambdaIR_Index=j;
%     end
%     if Lambda_UV==Global_tilt_Irr_2_2_12_13_5(j,2)
%         LambdaUV_Index=j;
%     end
% end


 %% Defining the optical and electrical properties of the used PV module
    U= LambdaIR_Index; %Index for Max. wavelength of IR not to block
%     O=1; % Factor to change the ambient temperauter, this is used to factor Taminet (assumable)to vary the reagion. 
    P=1; % P is assumed number of periods that solar irrandiance is almost same for these periods. 
    Index=0; % the index to take off from maximum Lambda IR that can be absorbed
    D=LambdaUV_Index;%1; % initial value that should be given to D (Index for Max. wavelength of UV to block) 
    Lamda = LambdaIR_Index; % 811; % index at which the maximum absorbed wavelength   
    IQE = 0.69005; % internal quantum efficiency of the cell
    RL = 0.356; % (Ohm) Resistive load (designed and experimentally measured)
    IL1(1,1) = 4;% (A) Load current (experimentally measure)
     
%     Lamda
%% Initializing the matrices

%      Io = NaN;
     wavelength=ones(1451,1);
     Tran = ones(1451,1);
     E=ones(1451,1);
     Photon_flux = ones(1451,1);
     Jph=ones(1451,1);
     Iph = ones(1451,1);
%      Voc = ones;
%      IL = ones;
%      VL = ones;
%      P_out = ones;
     frr =ones(1451,1);
     frr_poly = ones(1451,1);
%      Tm=ones(1,D);
%      hc_free=ones(1,D);
     

IL1(1,1) = 4;% (A) Load current (experimentally measure)

%% Finding the phtonic flux
Tran=Total_light_absorption_in_PV_cell_acrylic(1:U); % Total light transmission considering all layers and bounces through them
wavelength= 1e-9.*Global_tilt_Irr_2_2_12_13_5(1:U,2); % (m) wavelength
E = c.*h./wavelength; % (J) Energy per each wavelength
Photon_flux = Global_tilt_Irr_2_2_12_13_5(1:U,1)./E; % (photons/m2/nm/s) photon flux 

% for w=1 %:1:P*K/dt  
   w=1;

   
    Jph(D:Lamda)= q.*Tran(D:1:Lamda).*Photon_flux(D:Lamda).*IQE; %(Culomb/m2/nm/m/s = A/m2/nm)Short circuit current density 
    Iph(D:Lamda)= Aj.*1e-4.*Jph(D:Lamda); % (A/nm) Photo_generated current 


%% Photonic current per one cell
%    for z=D:1:Lamda
%     Jph(z,1)= q*Tran(z,1)*Photon_flux(z,1)*IQE; %(Culomb/m2/nm/m/s = A/m2/nm)Short circuit current density 
%     Iph (z,1) = Aj*1e-4*Jph(z,1); % (A/nm) Photo_generated current 
%    end
  
  Iph_total =0; % Intializing the current
  
%     for j=D:1:Lamda
        Iph_total = sum(Iph(D:Lamda,1)); % (A) Photonic current
%     end    
  
%% Calculating the input power term to cells
      Irr_total=0;
      
%       for j=D:1:Lamda
           E(D:1:Lamda)=h.*c./(wavelength(D:1:Lamda)); %(J) energy in each wavelength
           Irr_total= sum(Photon_flux(D:1:Lamda,1).*E(D:1:Lamda,1));% (W/m2/nm)Irradiance
%            Irr_total= frr(j,1)+Irr_total; % (W/m^2), this represents the integration to calculate total Irradiance for the specific wavelenght range. 
%       end

      Pin=Irr_total* A; % input power (W) to the module of M cells, each has Aj area in cm^2, A=M*Aj*1e-4    
      
%% Calculating the power input to the Polystyrene backing board
    Irr_poly=0;
    
%     for j=D:1:U % This represents the part of the board covered with cell
         E(D:1:U)=h.*c/(wavelength(D:1:U));
%          frr_poly(j,1)=Photon_flux(j,1)*Total_light_absorption_in_polystyren(j,1)*E(j,1);
         Irr_poly=sum(Photon_flux(D:1:U).*Total_light_absorption_in_polystyren(D:1:U).*E(D:1:U));
%     end

    Ppoly =Irr_poly*(A1-A); % (W) The power produced by the light absorbed by the backing Polystyrene plate

%% Calculating the saturation current using the refernece saturation current method
  
Io= Ior * (Tm_i/Tmr)^3*exp(q*Eg*(1/Tmr-1/Tm_i)/(k*N)); %(A) Saturation current as function of temperature
    
%% Calculating the output power consumed by the load
    nu=0.2; % solver constant
    %This loop is to solve for the load current numberically using Euler method 
    for s=1:1:10% s is counter reflects number of the solver steps needed to reach steady state current at a specific time step
        IL1(s+1) =nu*IL1(s)+(1-nu)*( N*k*Tm_i/(q*(RL/M+Rs))*log((Iph_total-IL1(s))/(Io)+1));
    end
%     IL1
    IL = IL1(end); % (V) Stabalized Output current passes the resistive load (0.3525 Ohm)in one time step
%     IL1 = IL1(end);  % setting a new initial load current for the next time step
    VL =  IL *RL; %Load voltage, or Iph_total-Io(w,1)*(exp(q*VL(w,1)/(N*k*Tm(w,1))-1)); %(A) Output current
   
%     P_out =real(VL*IL); %(W) Output power across the load 
   P_out=real(VL*IL);
   P_out=P_out(1);
   QQ=VL.*IL;
%  P_out(w,1)=0; % In case of open circuit condition

%% Calculating the output power in case of tracking the MPP
%      
%      Voc(w,1) = N*k*Tm(w,1)/q*log(Iph_total/Io(w,1)+1) ;  % (V) open circuit voltage
% 
%      Vocn(w,1)=q/(N*k*Tm(w,1))*Voc(w,1); % Normalized open circuit voltage
% 
%      Cff (w,1) = (Vocn(w,1)-log(Vocn(w,1)+0.72))/(Vocn(w,1)+1); % Filling factor
%               
%      rs=Rs/Rch; % ratio
%      
%      Cffn(w,1)=Cff(w,1)*(1-rs); % impact of the series resistance on the IV curve
%      
%     P_out(w,1)=M*Cffn(w,1)*Iph_total*Voc(w,1); % (W) output power of the module
      
%% Defining the terms of heat transfer


 
  hc_forced = 3.3*WS+6.5; % (W/(m^2.K)) Sharples windward relation to calculated hc_forced from the averaged wind speed 
    
  hc_free=1.31*(Tm_i-Tambient)^(1/3); % (W/(M^2.K)) Heat transfer coefficient due to air cooling on top surface and no wind
     
    Tsky=Tambient-deltT; % (K) Sky temperature
    %Tsky=Tambient; % (K) for overcast conditions
    Tground=Tambient; %(K) Ground temperature
     
%% Solving the 1st order nonlinear differenctial equation using Euler method
     Tm_f=Tm_i+dt.*(1/Cm*(segma*A*(((1+cos(Beta)/2)*e_sky_clear*(Tsky)^(4))+((1-cos(Beta))/2*e_g*(Tground)^(4))-(e_m*(Tm_i)^(4)))+ Ppoly + Pin -P_out-A.*(hc_forced^3+hc_free^3).^(1/3).*(Tm_i-Tambient))); %(K)Finding the module Temp
